simulink model "atrias_system"  (R2014a)
settings: Solver=FixedStepDiscrete  StartTime=0.0  StopTime=inf  FixedStep=sample_time  RelTol=1e-3
undefined symbols (not defined in the file): A_lpf_velocity, B1_lpf_velocity, B2_lpf_velocity, BOOM_MAX_ENCODER_TICKS, BOOM_PITCH_CAL_VALUE_RAD, BOOM_PITCH_CAL_VALUE_TICKS, BOOM_PITCH_ENCODER_RAD_PER_TICK, BOOM_ROLL_CAL_VALUE_RAD, BOOM_ROLL_CAL_VALUE_TICKS, BOOM_ROLL_ENCODER_RAD_PER_TICK, BOOM_YAW_ENCODER_RAD_PER_TICK, fcut_smooth, fcut_unwrap, gui_disable_cmd, gui_enable_cmd, gui_reset_cmd, HIP_ABS_ENCODER_RAD_PER_TICK, HIP_ABS_MAX_ENCODER_TICKS, HIP_INC_ENCODER_RAD_PER_TICK, HIP_INC_MAX_ENCODER_TICKS, HIP_MOTOR_CONSTANT, HIP_MTR_GEAR_RATIO, HIP_MTR_MAX_TORQUE, imu_daq_enable, INC_ENC_DIRS, INC_ENC_RAD_PER_TICK, k_sea, LEFT_HIP_CALIB_POS, LEFT_HIP_CALIB_VAL, LEFT_MOTOR_HIP_DIRECTION, LEG1_LEG_A_CALIB_VAL, LEG1_LEG_A_RAD_PER_CNT, LEG1_LEG_B_CALIB_VAL, LEG1_LEG_B_RAD_PER_CNT, LEG1_MOTOR_A_DIRECTION, LEG1_MOTOR_B_DIRECTION, LEG1_TRAN_A_CALIB_VAL, LEG1_TRAN_A_RAD_PER_CNT, LEG1_TRAN_B_CALIB_VAL, LEG1_TRAN_B_RAD_PER_CNT, LEG2_LEG_A_CALIB_VAL, LEG2_LEG_A_RAD_PER_CNT, LEG2_LEG_B_CALIB_VAL, LEG2_LEG_B_RAD_PER_CNT, LEG2_MOTOR_A_DIRECTION, LEG2_MOTOR_B_DIRECTION, LEG2_TRAN_A_CALIB_VAL, LEG2_TRAN_A_RAD_PER_CNT, LEG2_TRAN_B_CALIB_VAL, LEG2_TRAN_B_RAD_PER_CNT, LEG_A_CALIB_LOC, LEG_B_CALIB_LOC, LEG_MOTOR_CONSTANT, LEG_MTR_GEAR_RATIO, LEG_MTR_MAX_TORQUE, max_encoder_velocity, max_sensor_velocity, MEDULLA_ADC_MAX_VOLTS, MEDULLA_ADC_OFFSET_COUNTS, MEDULLA_STATE_ERROR ... (+15)
libraries: xpcethercatlib x174, simulink x22, dspswit3 x1
(part 4 of 4)

== matlab function atrias_system/DAQ/Leg Motor Observer ==
  data: u input double size=[1 6]; q input double; pos output double; rotor_vels input double; vel output; sample_time parameter double; k_sea parameter
function [pos,vel] = fcn(u, q, rotor_vels, sample_time, k_sea)
%#codegen

% Parameters:
%
%     u            Torque commands from the last cycle
%     q            The positional states vector (shouldn't be processed to remove dropouts -- this function does that as well)
%     rotor_vels   The current velocities computed using the incremental encoders in the motors
%     sample_time  The delta time between iterations (parameter defined in daq_params)
%     k_sea        The spring constants for the SEAs (parameter defined in sys_params)
%
% Return values
%
%     pos  A vector of motor positions (order defined below)
%     vel  A vector of motor velocities (order the same as pos)
%
% Order of state, y, etc... (matches rotor velocities):
%     back right
%     front right
%     back left
%     front left
%
% State: first row is position, second is velocity; each column is a
% different motor
%
% Much of the content of this function serves to reject bad absolute
% encoder signals. The 32-bit Renishaw encoders occasionally give bad data
% without setting any error bits. To filter these out, we compare the
% sensed position with the predicted (observed) position. We also look for
% repeated sensed positions, as that occurs when the encoder detects a bad
% reading.
%
% During absolute encoder dropouts, we fill in the missing position data
% using the incremental encoders. Other options for handling dropouts --
% which I have decided against -- include using a second observer design that
% relies only on the incremental encoder (only during dropouts) or just
% trusting the predicted state.


% Set up the system model. We only compute this on startup to save run time.
% Alternatively, we could've directly specified the discrete-time model,
% but I decided it was more readable to specify a continuous-time model and
% transform between the two in code.
persistent A
persistent B

if isempty(A) || isempty(B)
    % Form the continuous-time system model
    inertia = 3.0517; % Reflected moment of inertia (N*m*s^2/rad)
    A_cont  = [0 1; 0 0];
    B_cont  = [0; 1/inertia];
    
    % Translate the continuous-time system model to a discrete one. See
    % Wikipedia for the formula behind this.
    M = [A_cont B_cont; zeros(size(B_cont,2), size(A_cont,2) + size(B_cont,2))];
    M = expm(M * sample_time);
    A = M(1:size(A_cont, 1), 1:size(A_cont, 2));
    B = M(1:size(B_cont, 1), (size(A,2)+1):(size(A,2)+size(B_cont,2)));
end

% Observer gain matrix. Obtained via optimization on existing experimental
% data.
K = [ -0.014305247969510  0.010871733923180
      -7.301581788665865 -0.543374339802686 ];

% Retrieve the measured positions and velocities from the input vectors (in
% the order used by vel, pos, state, ...).
ypos = reshape(q([2 4 6 8]), 1, []);
yvel = reshape(rotor_vels,   1, []);
yleg = reshape(q([1 3 5 7]), 1, []);

% The model (and thus this function) begins running before EtherCAT data is
% available. We need to detect when data becomes available so we don't try
% to observe the state before then.
%
% These state variables are to detect the beginning of data acquisition
% (signaled by ypos changing)
persistent ypos_old
persistent has_data

if isempty(ypos_old) || isempty(has_data)
    ypos_old = ypos;
    has_data = false;
end

% Retain our current state estimate from cycle to cycle (this is the
% observer's memory)
persistent state

% Do initialization for the above state estimate
if isempty(state)
    % This value doesn't really matter; it is ignored while
    % has_data == false and gets reset when has_data becomes true.
    % We do need to get the size right, though, hence the use of ypos and
    % yvel
    state = [ypos; yvel];
end

% Check if we have data yet; if so, send dummy values.
% If we're just initializing now, reset the observer state to the sensed
% state
if ~has_data
    if all(ypos == ypos_old)
        % Not initialized yet; just output dummy data
        pos = pi * ones(1, 4);
        vel = zeros(1, 4);
        return
    else
        % We just got data for the first time! Initialize the observer state
        state    = [ypos; yvel];
        has_data = true;
    end
end

% Determine which position sensors have dropped out. The reasoning for this
% is described above (in the comments at the top of this file).
dropouts = (ypos == ypos_old) | (abs(ypos - state(1,:)) > .2);

% As mentioned above, we fake absolute encoder data during dropouts by
% using the rotor encoders. Assumption: no cycles are missed!
% Missed cycles will cause a drift in ypos for encoders that are currently
% dropped out (and the corresponding motor is moving).
% Assuming no encoders drop out for a long time, this drift will be
% negligible.
ypos(dropouts) = ypos_old(dropouts) + sample_time * yvel(dropouts);

% Update the "old" sensed positions for the next iteration.
ypos_old = ypos;

% Grab the torque commands for the relevant motors (same order as pos, vel,
% state, ...)
u = reshape(u([1 2 4 5]), 1, []);

% Compute the torques generated from the springs. We have no observer for
% the joint angles, so we just trust the sensors there. Since we don't need
% velocities (the damping constant is approximated by zero), the noise is
% negligible.
t_sprngs = k_sea .* (yleg - state(1,:));

% Run the discrete-time observer dynamics (finally!)
state = A * state + B * (u + t_sprngs) + K * (state - [ypos; yvel]);

% Set the function's return values from the current observer state
pos = state(1,:);
vel = state(2,:);
